simulink model "admittance_controller"  (R2021b)
settings: Solver=VariableStepAuto  StartTime=0.0  StopTime=10.0  RelTol=1e-3
values from neighbouring files (symbols this model uses):
  ddp_d = [0 0 0]'    [admittance_controller.m]
  dp_cd0 = [0 0 0]'    [admittance_controller.m]    (also in sim_admittance_controller.m; simulation_admittance_controller.m)
  dp_d = vel(4:6, :)'    [admittance_controller.m]
  f = [1 2 3]'    [admittance_controller.m]    (also in helpers.m = waitbar(0,"0","name","Simulating ODE 	ode_stats = @(t, y, fl; sim_admittance_controller.m = figure; sim_dampening.m = figure)
  Kd = eye(n)*kd    [admittance_controller.m]    (also in sim_admittance_controller.m = eye(3)*kd; sim_invdyn.m = eye(3)*50; simulation_admittance_controller.m = eye(3) * 4; simulation_invdyn.m = eye(3)*50)
  Kp = eye(n)*kp    [admittance_controller.m]    (also in sim_admittance_controller.m = eye(3)*kp; sim_invdyn.m = eye(3)*200; simulation_admittance_controller.m = eye(3) * 16; simulation_invdyn.m = eye(3)*200)
  Md = eye(n)*md    [admittance_controller.m]    (also in sim_admittance_controller.m = eye(3)*md; simulation_admittance_controller.m = eye(3) * 1)
  p_cd0 = [0 0 0]'    [admittance_controller.m]    (also in sim_admittance_controller.m; simulation_admittance_controller.m)
  p_d = [1 2 3]'    [admittance_controller.m]    (also in simulation_admittance_controller.m = timeseries(data, t))
settings Model: Creator=Martin  LastModifiedBy=Martin

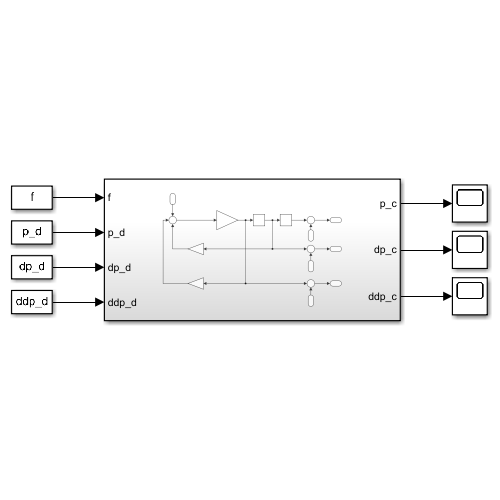
[thumbnail: Simulink's stored preview of the top-level diagram]
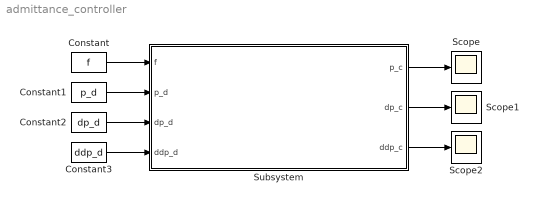
== system admittance_controller ==
  Constant : Constant  Value=f
  Constant1 : Constant  Value=p_d
  Constant2 : Constant  Value=dp_d
  Constant3 : Constant  Value=ddp_d
  Scope : Scope
  Scope1 : Scope
  Scope2 : Scope
  Subsystem : Subsystem
  wires:
  Constant/1 -> Subsystem/1(f)
  Constant1/1 -> Subsystem/2(p_d)
  Constant2/1 -> Subsystem/3(dp_d)
  Constant3/1 -> Subsystem/4(ddp_d)
  Subsystem/1(p_c) -> Scope/1
  Subsystem/2(dp_c) -> Scope1/1
  Subsystem/3(ddp_c) -> Scope2/1

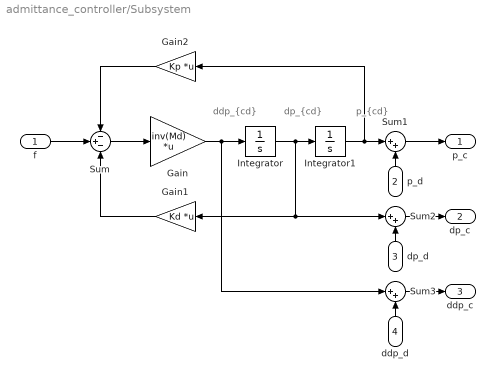
== system admittance_controller/Subsystem ==
  note: p_{cd}
  note: dp_{cd}
  note: ddp_{cd}
  f : Inport
  p_d : Inport  Port=2
  dp_d : Inport  Port=3
  ddp_d : Inport  Port=4
  Gain : Gain  Gain=inv(Md)  Multiplication=Matrix(K*u)
  Gain1 : Gain  Gain=Kd  Multiplication=Matrix(K*u)
  Gain2 : Gain  Gain=Kp  Multiplication=Matrix(K*u)
  Integrator : Integrator  InitialCondition=dp_cd0
  Integrator1 : Integrator  InitialCondition=p_cd0
  Sum : Sum  Inputs=-+-
  Sum1 : Sum  Inputs=|++
  Sum2 : Sum  Inputs=|++
  Sum3 : Sum  Inputs=|++
  p_c : Outport
  dp_c : Outport  Port=2
  ddp_c : Outport  Port=3
  wires:
  Sum2/1 -> dp_c/1
  Sum3/1 -> ddp_c/1
  Integrator/1 -> Gain1/1, Sum2/1, Integrator1/1
  Integrator1/1 -> Sum1/1, Gain2/1
  dp_d/1 -> Sum2/2
  Gain/1 -> Sum3/1, Integrator/1
  ddp_d/1 -> Sum3/2
  Sum1/1 -> p_c/1
  f/1 -> Sum/2
  p_d/1 -> Sum1/2
  Sum/1 -> Gain/1
  Gain2/1 -> Sum/1
  Gain1/1 -> Sum/3
